simulink model "closed_loop_pitch_autopilot"  (R2025b)
settings: Solver=VariableStepAuto  StartTime=0.0  StopTime=8  RelTol=1e-3
undefined symbols (not defined in the file): A, B, C, D
libraries: slpidlib x1
settings Model: Creator=shash  LastModifiedBy=shash

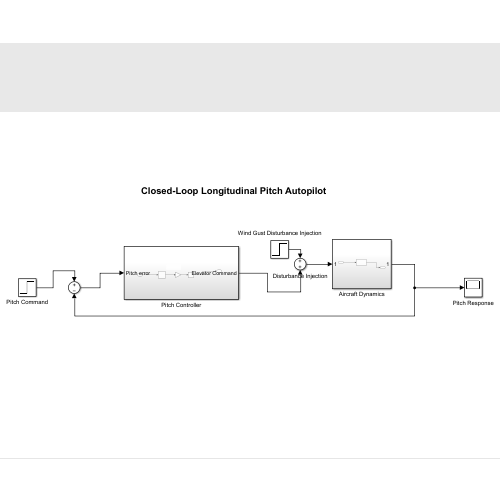
[thumbnail: Simulink's stored preview of the top-level diagram]
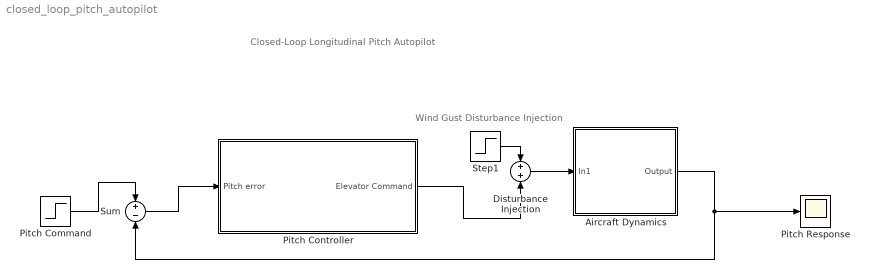
== system closed_loop_pitch_autopilot ==
  note: Wind Gust Disturbance Injection
  note: Closed-Loop Longitudinal Pitch Autopilot
  Aircraft Dynamics : Subsystem
  Disturbance Injection : Sum
  Pitch Command : Step  After=0.2  SampleTime=0
  Pitch Controller : Subsystem
  Pitch Response : Scope
      settings: ActiveDisplayYMinimum=-0.026841966567186935  ActiveDisplayYMaximum=0.24157769910468246
  Step1 : Step  Time=8  After=0.05  SampleTime=0
  Sum : Sum  Inputs=+-
  wires:
  Pitch Command/1 -> Sum/1
  Step1/1 -> Disturbance Injection/1
  Sum/1 -> Pitch Controller/1(Pitch error)
  Pitch Controller/1(Elevator Command) -> Disturbance Injection/2
  Aircraft Dynamics/1(Output) -> Sum/2, Pitch Response/1
  Disturbance Injection/1 -> Aircraft Dynamics/1(In1)

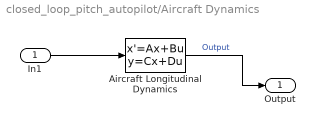
== system closed_loop_pitch_autopilot/Aircraft Dynamics ==
  In1 : Inport
  Aircraft Longitudinal Dynamics : StateSpace  A=A  B=B  C=C  D=D  InitialCondition=0
  Output : Outport
  wires:
  In1/1 -> Aircraft Longitudinal Dynamics/1
  Aircraft Longitudinal Dynamics/1 -> Output/1  "Output"

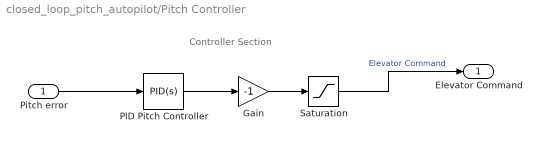
== system closed_loop_pitch_autopilot/Pitch Controller ==
  note: Controller Section
  Pitch error : Inport
  Gain : Gain  Gain=-1
  PID Pitch Controller : slpidlib/PID Controller  Controller=PID  Form=Parallel  TimeDomain=Continuous-time  UseExternalTs=off  SampleTime=-1  IntegratorMethod=Forward Euler  FilterMethod=Forward Euler  ControllerParametersSource=internal  P=1.5  I=0.2  UseKiTs=off  D=0.8  UseExternalDerivativeSource=off  N=100  UseFilter=on  TunerSelectOption=Transfer Function Based (PID Tuner App)  InitialConditionSource=internal  InitialConditionForIntegrator=0  InitialConditionForFilter=0  DifferentiatorICPrevScaledInput=0  ExternalReset=none  TrackingMode=off  Kt=1  LimitOutput=off  SatLimitsSource=internal  UpperSaturationLimit=inf  LowerSaturationLimit=-inf  LinearizeAsGain=on  AntiWindupMode=none  Kb=1  LimitIntegrator=off  UpperIntegratorSaturationLimit=inf  LowerIntegratorSaturationLimit=-inf  POutMin=[]  POutMax=[]  IOutMin=[]  IOutMax=[]  DOutMin=[]  DOutMax=[]  NOutMin=[]  NOutMax=[]  SumOutMin=[]  SumOutMax=[]  SaturationOutMin=[]  SaturationOutMax=[]  PParamMin=[]  PParamMax=[]  IParamMin=[]  IParamMax=[]  DParamMin=[]  DParamMax=[]  NParamMin=[]  NParamMax=[]  KbParamMin=[]  KbParamMax=[]  KtParamMin=[]  KtParamMax=[]  KbOutMin=[]  KbOutMax=[]  KtOutMin=[]  KtOutMax=[]  IntegratorOutMin=[]  IntegratorOutMax=[]  FilterOutMin=[]  FilterOutMax=[]  SumI1OutMin=[]  SumI1OutMax=[]  SumI2OutMin=[]  SumI2OutMax=[]  SumI3OutMin=[]  SumI3OutMax=[]  SumI4OutMin=[]  SumI4OutMax=[]  SumDOutMin=[]  SumDOutMax=[]  DifferentiatorOutMin=[]  DifferentiatorOutMax=[]  FilterDiffOutCoefMin=[]  FilterDiffOutCoefMax=[]  ReciprocalOutMin=[]  ReciprocalOutMax=[]  SumDenOutMin=[]  SumDenOutMax=[]  SumNumOutMin=[]  SumNumOutMax=[]  DivideOutMin=[]  DivideOutMax=[]  UdiffTsProdOutMin=[]  UdiffTsProdOutMax=[]  NTsProdOutMin=[]  NTsProdOutMax=[]  UintegralTsProdOutMin=[]  UintegralTsProdOutMax=[]  UngainTsProdOutMin=[]  UngainTsProdOutMax=[]  ClampingZeroOutDataTypeStr=Inherit: Inherit via back propagation  ClampingZeroOutMin=[]  ClampingZeroOutMax=[]  FilterDenConstantOutDataTypeStr=Inherit: Inherit via back propagation  FilterDenConstantOutMin=[]  FilterDenConstantOutMax=[]  PCopyOutDataTypeStr=Inherit: Inherit via back propagation  PCopyOutMin=[]  PCopyOutMax=[]  NCopyOutDataTypeStr=Inherit: Inherit via back propagation  NCopyOutMin=[]  NCopyOutMax=[]  IntegratorContinuousStateAttributes=''  IntegratorStateMustResolveToSignalObject=off  IntegratorRTWStateStorageClass=Auto  FilterContinuousStateAttributes=''  FilterStateMustResolveToSignalObject=off  FilterRTWStateStorageClass=Auto  ParallelPVariant=InternalParameters  IdealPVariant=Disabled  IVariant=InternalParameters  DVariant=InternalParameters  IntegratorVariant=Continuous  SatVariant=Disabled  AWVariant=Passthrough  PCopyVariant=Disabled  TRVariant=Disabled  FdbkBlocksVariant=Forward  IdealPFdbkVariant=Disabled  SatFdbkVariant=Disabled  DerivativeFilterVariant=ContFilter  NVariant=InternalParameters  NCopyVariant=Disabled  FilterICVariant=InternalICsFilter  IntegratorICVariant=InternalICs  ExternalResetVariant=Disabled  TRSumVariant=Passthrough  SumFdbkVariant=Disabled  SumVariant=Sum_PID  TsampFilterVariant=InternalTs  TsampNgainVariant=Passthrough  TsampIntegralVariant=Disabled_SignalSpec  ExternalSaturationOutDataTypeStr=Inherit: Same as second input  DerivativeSourceVariant=ErrorSignal  PreIntVariant=InternalPreInt
  Saturation : Saturate  UpperLimit=0.436  LowerLimit=-0.436
  Elevator Command : Outport
  wires:
  Pitch error/1 -> PID Pitch Controller/1
  Gain/1 -> Saturation/1
  PID Pitch Controller/1 -> Gain/1
  Saturation/1 -> Elevator Command/1  "Elevator Command"
